simulink model "view_wave_example_org"  (Simulink 10.0)
settings: Solver=FixedStepDiscrete  StartTime=0.0  StopTime=20  RelTol=1e-3
libraries: hdlsllib x1, simulink x1
settings Model: DataTypeOverride=Off  Creator=cchung  LastModifiedBy=bhisma
settings Model: LogicAnalyzerGraphicalSettings=|
  | {
  |   "cursors" : {
  |     "activeCursor" : 1,
  |     "lockedCursors" : [
  | 
  |     ],
  |     "startingCursor" : 0,
  |     "times" : [
  |       2,
  |       16
  |     ]
  |   },
  |   "global" : {
  |     "fontSize" : 12,
  |     "height" : 14
  |   },
  |   "panels" : [
  |     {
  |       "height" : 100,
  |       "startingTrace" : 0,
  |       "traces" : [
  |         {
  |           "signalId" : "de7ebb2f-2f7b-41dd-8cac-781ec53dba26",
  |           "type" : "wave"
  |         },
  |         {
  |           "signalId" : "7501e206-5046-48d9-b5db-df01969da4a0",
  |           "type" : "wave"
  |         },
  |         {
  |           "signalId" : "95e9138d-9991-4160-aa9e-9a7dd5c46aa6",
  |           "type" : "wave"
  |         },
  |         {
  |           "signalId" : "b293855a-55be-4f57-9423-70172f94ce6c",
  |           "type" : "wave"
  |         }
  |       ],
  |       "yOffset" : 0
  |     }
  |   ],
  |   "timeAxis" : {
  |     "pixelsPerSecond" : 29.65
  |   }
  | }
settings DataIOCC: LimitDataPoints=on  SaveOutput=off  SaveTime=off
settings OptimizationCC: BlockReduction=off  ConditionallyExecuteInputs=off  DefaultParameterBehavior=Inlined
settings DebuggingCC: AlgebraicLoopMsg=error  UnderspecifiedInitializationDetection=Simplified  MergeDetectMultiDrivingBlocksExec=error  SolverPrmCheckMsg=warning  SingleTaskRateTransMsg=error  StrictBusMsg=ErrorOnBusTreatedAsVector
settings HardwareCC: ProdHWDeviceType=ASIC/FPGA->ASIC/FPGA  ProdEqTarget=off
settings GRTTargetCC: GeneratePreprocessorConditionals=Disable all  CombineOutputUpdateFcns=on  GRTInterface=off
settings ConfigComp: CovExternalEMLEnable=off  CovSFcnEnable=off

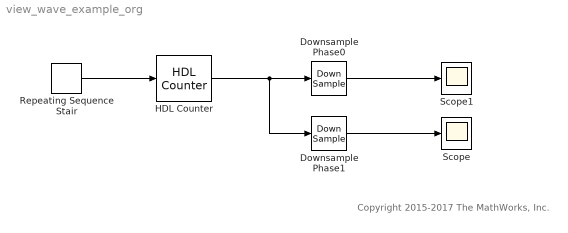
== system view_wave_example_org ==
  note: Copyright 2015-2017 The MathWorks, Inc.
  Downsample Phase0 : DownSample  RateOptions=Allow multirate processing
  Downsample Phase1 : DownSample  phase=1  RateOptions=Allow multirate processing
  HDL Counter : hdlsllib/Sources/HDL Counter  CountType=Free running  CountInit=0  CountStep=1  CountMax=25  CountFromType=Initial value  CountFrom=0  CountResetPort=off  CountLoadPort=off  CountEnbPort=on  CountDirPort=off  CountDataType=Unsigned  CountWordLen=6  CountFracLen=0  CountSampTime=1
      settings: SourceProductName=Simulink
  Repeating Sequence Stair : simulink/Sources/Repeating Sequence Stair  OutValues=[1 0 1 1 0].'  tsamp=1  OutMin=[]  OutMax=[]  OutDataTypeStr=fixdt('boolean')  OutputDataTypeScalingMode=Specify via dialog  OutDataType=fixdt('boolean')  ConRadixGroup=Best Precision: Vector-wise  OutScaling=[]
  Scope : Scope
  Scope1 : Scope
  wires:
  HDL Counter/1 -> Downsample Phase0/1, Downsample Phase1/1
  Repeating Sequence Stair/1 -> HDL Counter/1
  Downsample Phase1/1 -> Scope/1
  Downsample Phase0/1 -> Scope1/1
